simulink model "robot"  (R2014b)
settings: Solver=ode45  StartTime=0.0  StopTime=inf  RelTol=1e-3
values from neighbouring files (symbols this model uses):
  ts = 0.05    [analyze.m]
undefined symbols (not defined in the file or in its folder): dfilt, fdesignblkfcn, gcbh
libraries: arduino_io_lib x7, simulink x4, dsparch4 x2
settings Model: Creator=mike  LastModifiedBy=macbook
settings OptimizationCC: ExpressionDepthLimit=2147483647
settings DebuggingCC: UnderspecifiedInitializationDetection=Classic  MergeDetectMultiDrivingBlocksExec=none  StateNameClashWarn=warning

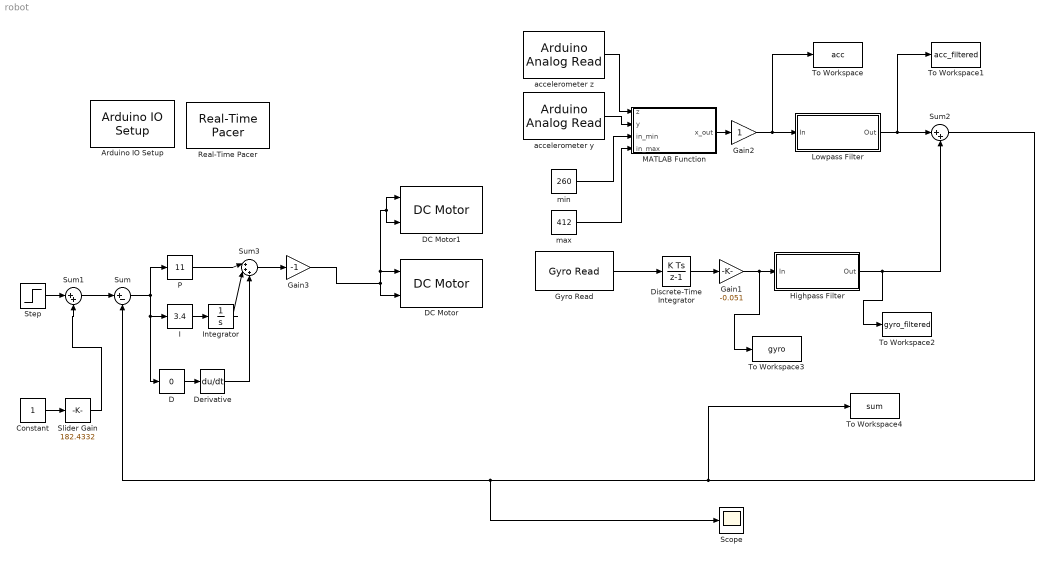
== system robot ==
  Arduino IO Setup : arduino_io_lib/Arduino IO Setup  Priority=3  arduinoVar=Temporary arduino variable: Arduino1  workspaceVarName=a  comPort=/dev/tty.usbmodem1411
  Constant : Constant
  D : simulink/Math Operations/Slider Gain  low=0  gain=0  high=7
  DC Motor : arduino_io_lib/DC Motor  arduinoVar=Temporary arduino variable: Arduino1  motorNum=3  sendOnChange=off  T=ts
  DC Motor1 : arduino_io_lib/DC Motor  arduinoVar=Temporary arduino variable: Arduino1  motorNum=4  sendOnChange=off  T=ts
  Derivative : Derivative
  Discrete-Time Integrator : DiscreteIntegrator  InitialConditionSetting=State (most efficient)  SampleTime=-1
  Gain1 : Gain  Gain=-0.051
  Gain2 : Gain  SampleTime=ts
  Gain3 : Gain  Gain=-1  SampleTime=ts
  Gyro Read : arduino_io_lib/Gyro Read  arduinoVar=Temporary arduino variable: Arduino1  axis=x  T=ts
  Highpass Filter : Subsystem  DialogController=fdesignblkfcn  InitFcn=fdesignblkfcn(gcbh, {'InitFcn'});  mask(Highpass Filter){}
      mask help: Design a highpass filter
      settings: CopyFcn=fdesignblkfcn(gcbh, {'CopyFcn'});
      mask Help: helpview(mapfilelocation('dsp'), 'dsphighpassfilter');
      mask Display: disp('Highpass')
  I : simulink/Math Operations/Slider Gain  low=0  gain=3.4  high=20
  Integrator : Integrator
  Lowpass Filter : Subsystem  DialogController=fdesignblkfcn  InitFcn=fdesignblkfcn(gcbh, {'InitFcn'});  mask(Lowpass Filter){}
      mask help: Design a lowpass filter
      settings: CopyFcn=fdesignblkfcn(gcbh, {'CopyFcn'});
      mask Help: helpview(mapfilelocation('dsp'), 'dsplowpassfilter');
      mask Display: disp('Lowpass')
  MATLAB Function : MATLAB Function  TreatAsAtomicUnit=on
  P : simulink/Math Operations/Slider Gain  low=1  gain=11  high=11
  Real-Time Pacer : arduino_io_lib/Real-Time Pacer  simTimePerRealTime=1
  Scope : Scope
      settings: YMin=40  YMax=220
  Slider Gain : simulink/Math Operations/Slider Gain  low=160  gain=182.4332  high=360
  Step : Step  Time=0  After=0  SampleTime=0
  Sum : Sum  Inputs=|+-
  Sum1 : Sum  Inputs=|++
  Sum2 : Sum  Inputs=|++
  Sum3 : Sum  Inputs=|+++
  To Workspace : ToWorkspace  VariableName=acc  SaveFormat=Timeseries  SampleTime=-1
  To Workspace1 : ToWorkspace  VariableName=acc_filtered  SaveFormat=Timeseries  SampleTime=-1
  To Workspace2 : ToWorkspace  VariableName=gyro_filtered  SaveFormat=Timeseries  SampleTime=-1
  To Workspace3 : ToWorkspace  VariableName=gyro  SaveFormat=Timeseries  SampleTime=-1
  To Workspace4 : ToWorkspace  VariableName=sum  SaveFormat=Timeseries  SampleTime=-1
  accelerometer y : arduino_io_lib/Arduino Analog Read  arduinoVar=Temporary arduino variable: Arduino1  arduinoPin=1  T=ts
  "accelerometer z " : arduino_io_lib/Arduino Analog Read  arduinoVar=Temporary arduino variable: Arduino1  arduinoPin=0  T=ts
  max : Constant  Value=412
  min : Constant  Value=260
  wires:
  Step/1 -> Sum1/1
  Sum/1 -> D/1, I/1, P/1
  Gain3/1 -> DC Motor1/1, DC Motor1/2, DC Motor/1, DC Motor/2
  Constant/1 -> Slider Gain/1
  Slider Gain/1 -> Sum1/2
  Sum1/1 -> Sum/1
  Gyro Read/1 -> Discrete-Time Integrator/1
  Discrete-Time Integrator/1 -> Gain1/1
  "accelerometer z "/1 -> MATLAB Function/1(z)
  accelerometer y/1 -> MATLAB Function/2(y)
  min/1 -> MATLAB Function/3(in_min)
  max/1 -> MATLAB Function/4(in_max)
  Lowpass Filter/1(Out) -> To Workspace1/1, Sum2/1
  MATLAB Function/1(x_out) -> Gain2/1
  Highpass Filter/1(Out) -> To Workspace2/1, Sum2/2
  Gain1/1 -> To Workspace3/1, Highpass Filter/1(In)
  Gain2/1 -> To Workspace/1, Lowpass Filter/1(In)
  I/1 -> Integrator/1
  Integrator/1 -> Sum3/2
  P/1 -> Sum3/1
  D/1 -> Derivative/1
  Derivative/1 -> Sum3/3
  Sum3/1 -> Gain3/1
  Sum2/1 -> To Workspace4/1, Scope/1, Sum/2

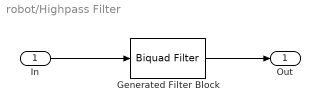
== system robot/Highpass Filter ==
  In : Inport
  Generated Filter Block : dsparch4/Biquad Filter  Tag=BlockMethodSubSystem  IIRFiltStruct=Direct form II  CoeffSource=Specify via dialog  BiQuadCoeffs=[2 -2 0 1 -0.853644417025241853 0]  a0Flag=Warning  IC=0  ICnum=0  ICden=0  InputProcessing=Columns as channels (frame based)  denAccumFracLength=30  denProdOutputFracLength=30  secondMemoryFracLength=15  roundingMode=Floor  overflowMode=off  ScaleValues=[0.146355582974758147;3.16633704596178411]  optimizeScaleValues=off  ScaleValueMode=Specify via input port (g)  scaleValueFracLength=14  FilterSource=Specify via dialog  dfiltObjectName=dfilt.df2tsos([1 0.3 0.4],[1 0.1 0.2])
  Out : Outport
  wires:
  Generated Filter Block/1 -> Out/1
  In/1 -> Generated Filter Block/1

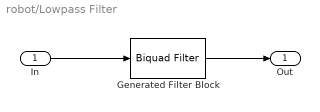
== system robot/Lowpass Filter ==
  In : Inport
  Generated Filter Block : dsparch4/Biquad Filter  Tag=BlockMethodSubSystem  IIRFiltStruct=Direct form II  CoeffSource=Specify via dialog  BiQuadCoeffs=[0.499999999999999889 0.499999999999999889 0 1 -0.883665323160146121 0]  a0Flag=Warning  IC=0  ICnum=0  ICden=0  InputProcessing=Columns as channels (frame based)  denAccumFracLength=30  denProdOutputFracLength=30  secondMemoryFracLength=15  roundingMode=Floor  overflowMode=off  ScaleValues=[0.116334676839853893;1]  optimizeScaleValues=off  ScaleValueMode=Specify via input port (g)  scaleValueFracLength=14  FilterSource=Specify via dialog  dfiltObjectName=dfilt.df2tsos([1 0.3 0.4],[1 0.1 0.2])
  Out : Outport
  wires:
  In/1 -> Generated Filter Block/1
  Generated Filter Block/1 -> Out/1

== matlab function robot/MATLAB Function ==
  data: z input; y input; in_min input; in_max input; x_out output
function x_out = fcn(z,y,in_min,in_max)
%#codegen

out_min = -90;
out_max = 90;

z_scaled = (z - in_min) * (out_max - out_min) / (in_max - in_min) + out_min;
y_scaled = (y - in_min) * (out_max - out_min) / (in_max - in_min) + out_min;

x_out = (180/pi)*( (atan2(-y_scaled, -z_scaled) + pi));
